simulink model "Turbine_model"  (R2023a)
settings: Solver=VariableStepAuto  StartTime=0.0  StopTime=10.0  RelTol=1e-3
values from neighbouring files (symbols this model uses):
  d_base = data_DF(13)    [find_dfig_state_initial_conditions.m]    (also in test_dfig.m = 5)
  d_Beta = 0    [dfig_smib_main.m]    (also in find_dfig_state_initial_conditions.m; test_dfig.m)
  d_bl = 40.05    [dfig_smib_main.m]    (also in find_dfig_state_initial_conditions.m; test_dfig.m)
  d_Cdc = 2    [dfig_smib_main.m]    (also in find_dfig_state_initial_conditions.m; test_dfig.m)
  d_Cf = 0.0150    (= 0.015)    [dfig_smib_main.m]    (also in find_dfig_state_initial_conditions.m = d_FLTR(6); test_dfig.m)
  d_ctg = 0.01    [dfig_smib_main.m]    (also in find_dfig_state_initial_conditions.m = data_DF(10); test_dfig.m)
  d_esd = -d_Kmrr.*d_ws.*(d_Lrr.*d_irq + d_Lm.*d_isq)    [find_dfig_state_initial_conditions.m]
  d_esq = d_Kmrr.*d_ws.*(d_Lrr.*d_ird + d_Lm.*d_isd)    [find_dfig_state_initial_conditions.m]
  d_iid = 0.0024    [dfig_smib_main.m]    (also in test_dfig.m)
  d_iiq = xdfig(:,7)    [find_dfig_state_initial_conditions.m]
  d_isd = 0.2454    [dfig_smib_main.m]    (also in find_dfig_state_initial_conditions.m = xdfig(:,2); test_dfig.m)
  d_isq = xdfig(:,1)    [find_dfig_state_initial_conditions.m]
  d_Kmrr = d_Lm/d_Lrr    (= 0.98517314418)    [dfig_smib_main.m]    (also in find_dfig_state_initial_conditions.m = d_Lm/d_Lrr; test_dfig.m)
  d_kopt = 1    [dfig_smib_main.m]    (also in find_dfig_state_initial_conditions.m = data_DF(8); test_dfig.m)
  d_ktg = 0.3    [dfig_smib_main.m]    (also in find_dfig_state_initial_conditions.m = data_DF(9); test_dfig.m)
  d_Lg = 0.0033    [dfig_smib_main.m]    (also in find_dfig_state_initial_conditions.m = d_FLTR(5); test_dfig.m)
  d_Li = 0.1667    [dfig_smib_main.m]    (also in find_dfig_state_initial_conditions.m = d_FLTR(4); test_dfig.m)
  d_Lm = 4    [dfig_smib_main.m]    (also in find_dfig_state_initial_conditions.m = data_DF(3); test_dfig.m)
  d_MSC_IL1_iv = 0.0389    [dfig_smib_main.m]    (also in test_dfig.m)
  d_MSC_IL1_ki = -3    [dfig_smib_main.m]    (also in find_dfig_state_initial_conditions.m; test_dfig.m)
  d_MSC_IL1_kp = -0.23    [dfig_smib_main.m]    (also in find_dfig_state_initial_conditions.m; test_dfig.m)
  d_MSC_IL2_ki = -3    [dfig_smib_main.m]    (also in find_dfig_state_initial_conditions.m; test_dfig.m)
  d_MSC_IL2_kp = -0.23    [dfig_smib_main.m]    (also in find_dfig_state_initial_conditions.m; test_dfig.m)
  d_MSC_OL1_iv = -0.8927    [dfig_smib_main.m]    (also in test_dfig.m)
  d_MSC_OL1_ki = -60    [dfig_smib_main.m]    (also in find_dfig_state_initial_conditions.m; test_dfig.m)
  d_MSC_OL1_kp = 0    [dfig_smib_main.m]    (also in find_dfig_state_initial_conditions.m; test_dfig.m)
  d_MSC_OL2_ki = 90    [dfig_smib_main.m]    (also in find_dfig_state_initial_conditions.m; test_dfig.m)
  d_MSC_OL2_kp = 0    [dfig_smib_main.m]    (also in find_dfig_state_initial_conditions.m; test_dfig.m)
  d_Qs = 0.1    [dfig_smib_main.m]    (also in find_dfig_state_initial_conditions.m = Qdfiq; test_dfig.m)
  d_R1 = d_Rs + d_R2    (= 0.0103381136821)    [dfig_smib_main.m]    (also in find_dfig_state_initial_conditions.m = d_Rs + d_R2; test_dfig.m)
  d_R2 = d_Kmrr^2*d_Rr    (= 0.00533811368208)    [dfig_smib_main.m]    (also in find_dfig_state_initial_conditions.m = d_Kmrr^2*d_Rr; test_dfig.m)
  d_Rc = 0.7333    [dfig_smib_main.m]    (also in find_dfig_state_initial_conditions.m = d_FLTR(3); test_dfig.m)
  d_Rg = 0.0    (= 0)    [dfig_smib_main.m]    (also in find_dfig_state_initial_conditions.m; test_dfig.m)
  d_Ri = 0.0    (= 0)    [dfig_smib_main.m]    (also in find_dfig_state_initial_conditions.m; test_dfig.m)
  d_Tr = d_Lrr/d_Rr    [find_dfig_state_initial_conditions.m]
  d_Ts = 0.9385    [dfig_smib_main.m]    (also in find_dfig_state_initial_conditions.m = dTg; test_dfig.m)
  d_vcq = 0.9837    [dfig_smib_main.m]    (also in find_dfig_state_initial_conditions.m = xdfig(:,13); test_dfig.m)
  d_VDC = 1.5    [dfig_smib_main.m]    (also in test_dfig.m)
  d_vrd = 0.0154    [dfig_smib_main.m]    (also in test_dfig.m)
  d_vrq = 0.0357    [dfig_smib_main.m]    (also in test_dfig.m)
  d_vw = 14.5316    [dfig_smib_main.m]    (also in test_dfig.m)
  d_welb = 2*pi*50    (= 314.159265359)    [find_dfig_state_initial_conditions.m]    (also in test_dfig.m)
  d_ws = 1.0    (= 1)    [find_dfig_state_initial_conditions.m]    (also in test_dfig.m = 314.159265359)
  d_wtrated = 3.0337    [dfig_smib_main.m]    (also in find_dfig_state_initial_conditions.m; test_dfig.m)
  d_Xm = d_Lm    (= 4)    [dfig_smib_main.m]    (also in find_dfig_state_initial_conditions.m = d_Lm; test_dfig.m)
  rho = 1.225    [dfig_smib_main.m]    (also in find_dfig_state_initial_conditions.m; test_dfig.m)
undefined symbols (not defined in the file or in its folder): d_Lsd, d_p, d_vdc, d_w, d_wb
settings Model: Creator=rufar  LastModifiedBy=rufar

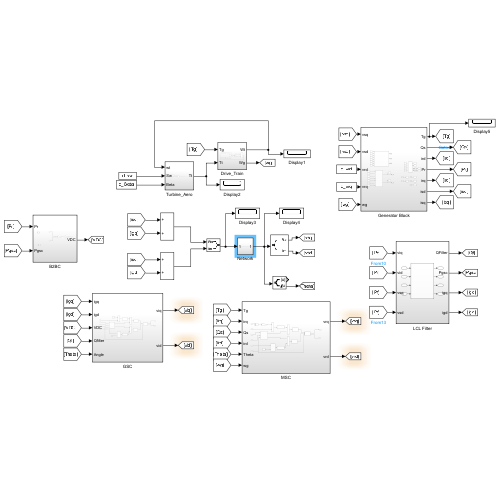
[thumbnail: Simulink's stored preview of the top-level diagram]
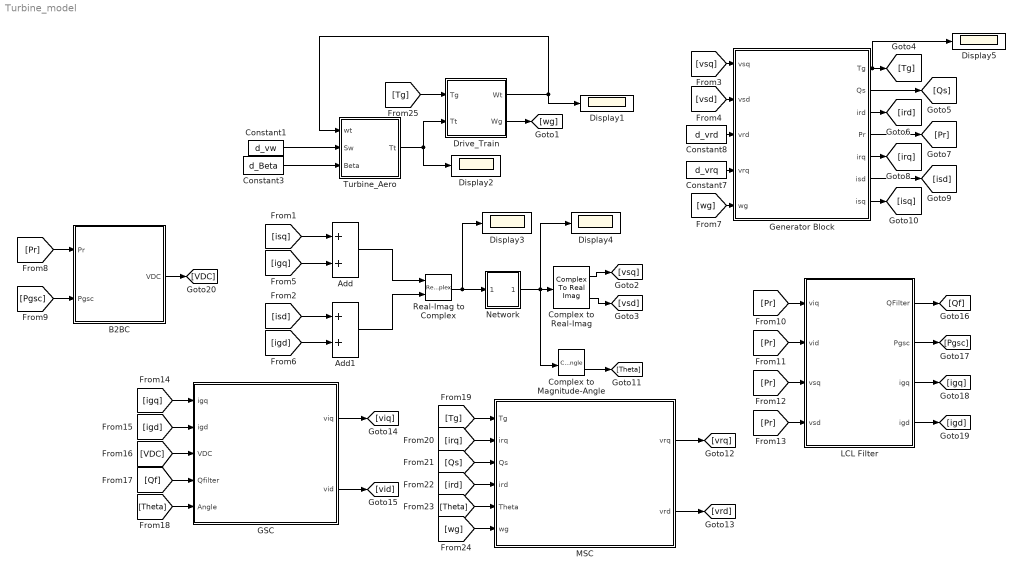
== system Turbine_model ==
  Add : Sum
  Add1 : Sum
  B2BC : Subsystem
  Complex to Magnitude-Angle : ComplexToMagnitudeAngle
  Complex to Real-Imag : ComplexToRealImag
  Constant1 : Constant  Value=d_vw
  Constant3 : Constant  Value=d_Beta
  Constant7 : Constant  Value=d_vrq
  Constant8 : Constant  Value=d_vrd
  Display{1..5} (5 alike) : Scope
  Drive_Train : Subsystem
  GSC : Subsystem
  Generator Block : Subsystem
  LCL Filter : Subsystem
  MSC : Subsystem
  Network : Subsystem
  Real-Imag to Complex : RealImagToComplex
  Turbine_Aero : Subsystem
  wires:
  Constant1/1 -> Turbine_Aero/2(Sw)
  Constant3/1 -> Turbine_Aero/3(Beta)
  Drive_Train/1(Wt) -> Display1/1, Turbine_Aero/1(wt)
  [Tg] -> Drive_Train/1(Tg)
  Drive_Train/2(Wg) -> [wg]
  Turbine_Aero/1(Tt) -> Drive_Train/2(Tt), Display2/1
  [igq] -> Add/2
  [igd] -> Add1/2
  Add/1 -> Real-Imag to Complex/1
  Add1/1 -> Real-Imag to Complex/2
  Real-Imag to Complex/1 -> Network/1(In1), Display3/1
  Complex to Real-Imag/1 -> [vsq]
  Complex to Real-Imag/2 -> [vsd]
  [isq] -> Add/1
  [isd] -> Add1/1
  [vsq] -> Generator Block/1(vsq)
  [vsd] -> Generator Block/2(vsd)
  [wg] -> Generator Block/5(wg)
  Constant7/1 -> Generator Block/4(vrq)
  Constant8/1 -> Generator Block/3(vrd)
  Generator Block/1(Tg) -> Display5/1, [Tg]
  Generator Block/2(Qs) -> [Qs]
  Generator Block/3(ird) -> [ird]
  Generator Block/4(Pr) -> [Pr]
  Generator Block/5(irq) -> [irq]
  Generator Block/6(isd) -> [isd]
  Generator Block/7(isq) -> [isq]
  Network/1(Out1) -> Complex to Magnitude-Angle/1, Display4/1, Complex to Real-Imag/1
  Complex to Magnitude-Angle/2 -> [Theta]
  [Pr] -> B2BC/1(Pr)
  [Pgsc] -> B2BC/2(Pgsc)
  [Pr] -> LCL Filter/1(viq)
  [Pr] -> LCL Filter/2(vid)
  [Pr] -> LCL Filter/3(vsq)
  [Pr] -> LCL Filter/4(vsd)
  [igq] -> GSC/1(igq)
  [igd] -> GSC/2(igd)
  [VDC] -> GSC/3(VDC)
  [Qf] -> GSC/4(Qfilter)
  [Theta] -> GSC/5(Angle)
  [Tg] -> MSC/1(Tg)
  [irq] -> MSC/2(irq)
  [Qs] -> MSC/3(Qs)
  [ird] -> MSC/4(ird)
  [Theta] -> MSC/5(Theta)
  [wg] -> MSC/6(wg)
  MSC/1(vrq) -> [vrq]
  MSC/2(vrd) -> [vrd]
  GSC/2(vid) -> [vid]
  GSC/1(viq) -> [viq]
  LCL Filter/1(QFilter) -> [Qf]
  LCL Filter/3(igq) -> [igq]
  LCL Filter/4(igd) -> [igd]
  LCL Filter/2(Pgsc) -> [Pgsc]
  B2BC/1(VDC) -> [VDC]

== system Turbine_model/B2BC ==
  Pr : Inport
  Pgsc : Inport  Port=2
  Add : Sum
  Add1 : Sum  Inputs=+-
  Gain : Gain  Gain=d_Cdc/d_p
  Gain1 : Gain  Gain=1/d_vdc
  Product : Product
  VDC : Outport
  wires:
  Gain/1 -> VDC/1
  Pr/1 -> Add1/1
  Pgsc/1 -> Add1/2
  Add1/1 -> Gain1/1
  Gain1/1 -> Gain/1

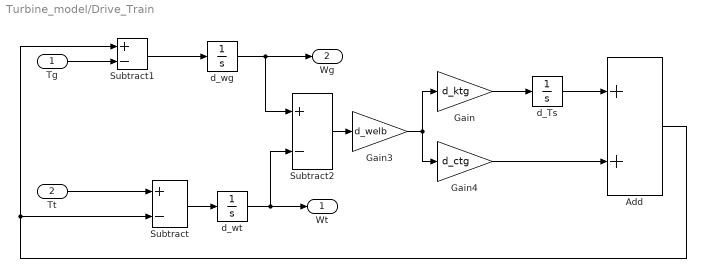
== system Turbine_model/Drive_Train ==
  Tg : Inport
  Tt : Inport  Port=2
  Add : Sum
  Gain : Gain  Gain=d_ktg
  Gain3 : Gain  Gain=d_welb
  Gain4 : Gain  Gain=d_ctg
  Subtract : Sum  Inputs=+-
  Subtract1 : Sum  Inputs=+-
  Subtract2 : Sum  Inputs=+-
  d_Ts : Integrator  InitialCondition=d_Ts
  d_wg : Integrator
  d_wt : Integrator
  Wt : Outport
  Wg : Outport  Port=2
  wires:
  Subtract1/1 -> d_wg/1
  Tg/1 -> Subtract1/2
  Gain3/1 -> Gain/1, Gain4/1
  d_wt/1 -> Wt/1, Subtract2/2
  Add/1 -> Subtract1/1, Subtract/2
  d_Ts/1 -> Add/1
  d_wg/1 -> Wg/1, Subtract2/1
  Gain/1 -> d_Ts/1
  Subtract2/1 -> Gain3/1
  Tt/1 -> Subtract/1
  Subtract/1 -> d_wt/1
  Gain4/1 -> Add/2

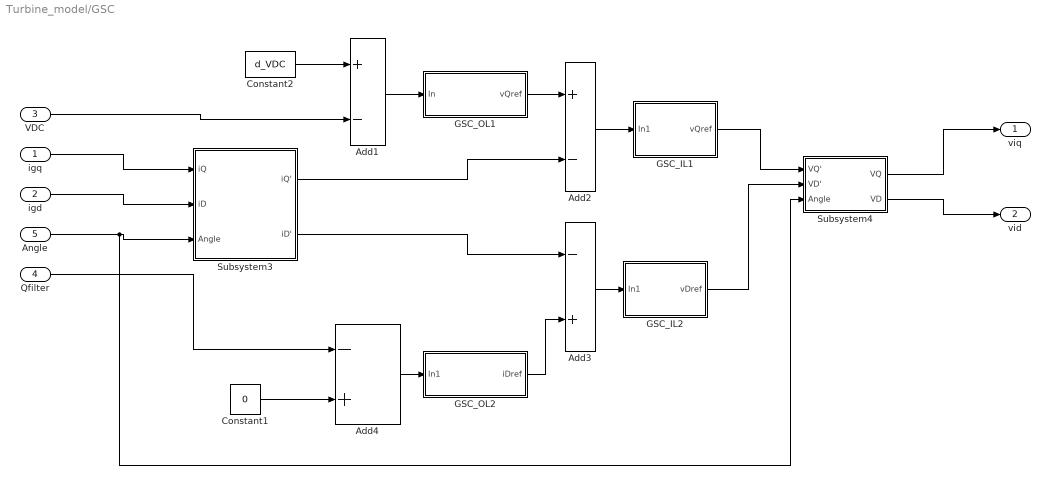
== system Turbine_model/GSC ==
  igq : Inport
  igd : Inport  Port=2
  VDC : Inport  Port=3
  Qfilter : Inport  Port=4
  Angle : Inport  Port=5
  Add1 : Sum  Inputs=+-
  Add2 : Sum  Inputs=+-
  Add3 : Sum  Inputs=-+
  Add4 : Sum  Inputs=-+
  Constant1 : Constant  Value=0
  Constant2 : Constant  Value=d_VDC
  GSC_IL1 : Subsystem
  GSC_IL2 : Subsystem
  GSC_OL1 : Subsystem
  GSC_OL2 : Subsystem
  Subsystem3 : Subsystem
  Subsystem4 : Subsystem
  viq : Outport
  vid : Outport  Port=2
  wires:
  Add2/1 -> GSC_IL1/1(In1)
  Constant1/1 -> Add4/2
  GSC_IL2/1(vDref) -> Subsystem4/2(VD')
  GSC_OL2/1(iDref) -> Add3/2
  Subsystem3/2(iD') -> Add3/1
  Add3/1 -> GSC_IL2/1(In1)
  GSC_IL1/1(vQref) -> Subsystem4/1(VQ')
  Add4/1 -> GSC_OL2/1(In1)
  Subsystem3/1(iQ') -> Add2/2
  GSC_OL1/1(vQref) -> Add2/1
  Add1/1 -> GSC_OL1/1(In)
  Constant2/1 -> Add1/1
  Qfilter/1 -> Add4/1
  VDC/1 -> Add1/2
  igq/1 -> Subsystem3/1(iQ)
  igd/1 -> Subsystem3/2(iD)
  Angle/1 -> Subsystem4/3(Angle), Subsystem3/3(Angle)
  Subsystem4/1(VQ) -> viq/1
  Subsystem4/2(VD) -> vid/1

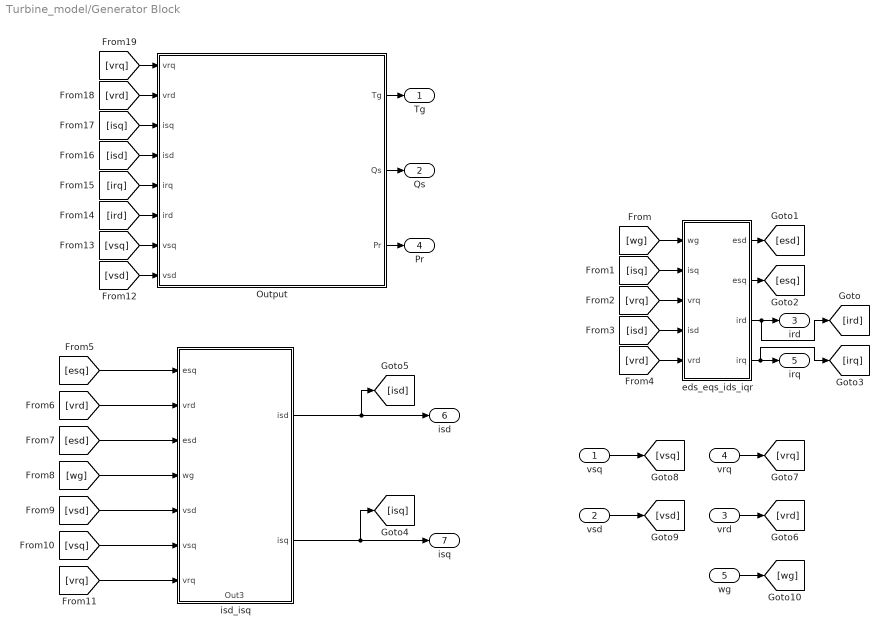
== system Turbine_model/Generator Block ==
  vsq : Inport
  vsd : Inport  Port=2
  vrd : Inport  Port=3
  vrq : Inport  Port=4
  wg : Inport  Port=5
  Output : Subsystem
  eds_eqs_ids_iqr : Subsystem
  isd_isq : Subsystem
      settings: PortSchema="{\"entries\":[{\"content\":{\"sides\":[{\"content\":{\"connectorIds\":[\"In1\",\"In2\",\"In3\",\"In4\",\"In5\",\"In6\",\"In7\"]},\"type\":\"ConnectorPlacement.EquallySpacedRectSide\",\"uuid\":\"c5511185-da93-4ae8-88f6-29fd087d6847\"},{\"content\":{\"connectorIds\":[\"Out1\",\"Out2\"],\"side\":\"RIGHT\"},\"type\":\"ConnectorPlacement.EquallySpacedRectSide\",\"uuid\":\"8a51c219-b932-42a4-96d0-f80c9d1d2533\"},{\"content\":{\"side\":\"TOP\"},\"type\":\"ConnectorPlacement.EquallySpacedRectSide\",\"uuid\":\"7f9cc9f4-8f0b-466b-9f07-e1686915bf69\"},{\"content\":{\"connectorIds\":[\"Out3\"],\"side\":\"BOTTOM\"},\"type\":\"ConnectorPlacement.EquallySpacedRectSide\",\"uuid\":\"e11d6ee8-9751-46c5-ba7a-4a49ef168c79\"}]},\"type\":\"ConnectorPlacement.EquallySpacedConnector\",\"uuid\":\"445fd2cf-43b7-4f11-a009-da067b61af35\"}],\"packageUris\":[\"http://schema.mathworks.com/mf0/Connector/R2020b\"],\"version\":\"1.0\"}"
  Tg : Outport
  Qs : Outport  Port=2
  ird : Outport  Port=3
  Pr : Outport  Port=4
  irq : Outport  Port=5
  isd : Outport  Port=6
  isq : Outport  Port=7
  wires:
  [isd] -> eds_eqs_ids_iqr/4(isd)
  [esq] -> isd_isq/1(esq)
  [wg] -> isd_isq/4(wg)
  [vrq] -> isd_isq/7(vrq)
  Output/1(Tg) -> Tg/1
  isd_isq/1(isd) -> [isd], isd/1
  isd_isq/2("isq ") -> [isq], isq/1
  [irq] -> Output/5(irq)
  [vrd] -> isd_isq/2(vrd)
  Output/3(Pr) -> Pr/1
  eds_eqs_ids_iqr/1(esd) -> [esd]
  [vrq] -> eds_eqs_ids_iqr/3(vrq)
  [isd] -> Output/4(isd)
  eds_eqs_ids_iqr/4(irq) -> [irq], irq/1
  [vsd] -> isd_isq/5(vsd)
  [esd] -> isd_isq/3(esd)
  [isq] -> eds_eqs_ids_iqr/2(isq)
  [vrd] -> eds_eqs_ids_iqr/5(vrd)
  [vsq] -> isd_isq/6(vsq)
  eds_eqs_ids_iqr/2(esq) -> [esq]
  [isq] -> Output/3(isq)
  [ird] -> Output/6(ird)
  [vsq] -> Output/7(vsq)
  [vsd] -> Output/8(vsd)
  [vrd] -> Output/2(vrd)
  Output/2(Qs) -> Qs/1
  [vrq] -> Output/1(vrq)
  [wg] -> eds_eqs_ids_iqr/1(wg)
  eds_eqs_ids_iqr/3(ird) -> [ird], ird/1
  vsq/1 -> [vsq]
  vsd/1 -> [vsd]
  vrd/1 -> [vrd]
  vrq/1 -> [vrq]
  wg/1 -> [wg]

== system Turbine_model/LCL Filter ==
  viq : Inport
  vid : Inport  Port=2
  vsq : Inport  Port=3
  vsd : Inport  Port=4
  LCL Filter : Subsystem
  QFilter : Outport
  Pgsc : Outport  Port=2
  igq : Outport  Port=3
  igd : Outport  Port=4
  wires:
  viq/1 -> LCL Filter/1(viq)
  LCL Filter/2(Pgsc) -> Pgsc/1
  vsd/1 -> LCL Filter/4(vsd)
  vsq/1 -> LCL Filter/3(vsq)
  vid/1 -> LCL Filter/2(vid)
  LCL Filter/1(QFilter) -> QFilter/1
  LCL Filter/3(igq) -> igq/1
  LCL Filter/4(igd) -> igd/1

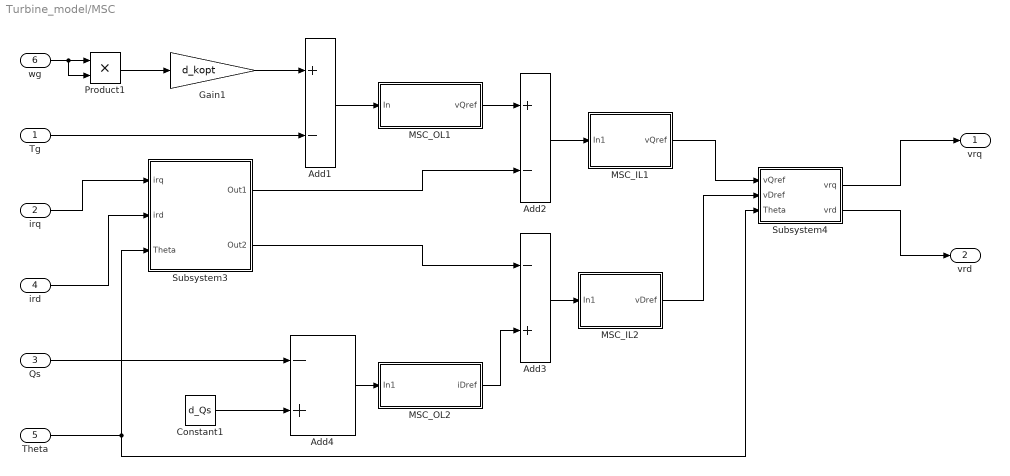
== system Turbine_model/MSC ==
  Tg : Inport
  irq : Inport  Port=2
  Qs : Inport  Port=3
  ird : Inport  Port=4
  Theta : Inport  Port=5
  wg : Inport  Port=6
  Add1 : Sum  Inputs=+-
  Add2 : Sum  Inputs=+-
  Add3 : Sum  Inputs=-+
  Add4 : Sum  Inputs=-+
  Constant1 : Constant  Value=d_Qs
  Gain1 : Gain  Gain=d_kopt
  MSC_IL1 : Subsystem
  MSC_IL2 : Subsystem
  MSC_OL1 : Subsystem
  MSC_OL2 : Subsystem
  Product1 : Product
  Subsystem3 : Subsystem
  Subsystem4 : Subsystem
  vrq : Outport
  vrd : Outport  Port=2
  wires:
  wg/1 -> Product1/2, Product1/1
  Product1/1 -> Gain1/1
  Gain1/1 -> Add1/1
  Tg/1 -> Add1/2
  Add1/1 -> MSC_OL1/1(In)
  MSC_OL1/1(vQref) -> Add2/1
  irq/1 -> Subsystem3/1(irq)
  ird/1 -> Subsystem3/2(ird)
  Theta/1 -> Subsystem4/3(Theta), Subsystem3/3(Theta)
  Subsystem3/1(Out1) -> Add2/2
  Qs/1 -> Add4/1
  Constant1/1 -> Add4/2
  Subsystem4/1(vrq) -> vrq/1
  Subsystem3/2(Out2) -> Add3/1
  Subsystem4/2(vrd) -> vrd/1
  MSC_IL2/1(vDref) -> Subsystem4/2(vDref)
  MSC_IL1/1(vQref) -> Subsystem4/1(vQref)
  Add3/1 -> MSC_IL2/1(In1)
  MSC_OL2/1(iDref) -> Add3/2
  Add2/1 -> MSC_IL1/1(In1)
  Add4/1 -> MSC_OL2/1(In1)

== system Turbine_model/Network ==
  In1 : Inport
  Out1 : Outport
  wires:
  In1/1 -> Out1/1

== system Turbine_model/Turbine_Aero ==
  wt : Inport
  Sw : Inport  Port=2
  Beta : Inport  Port=3
  Subsystem : Subsystem
  Tt : Outport
  wires:
  Beta/1 -> Subsystem/3(Beta)
  Subsystem/1(Tt) -> Tt/1
  Sw/1 -> Subsystem/2(Sw)
  wt/1 -> Subsystem/1(wt)

== system Turbine_model/GSC/GSC_IL1 ==
  In1 : Inport
  Gain1 : Gain  Gain=d_MSC_IL1_ki
  Gain2 : Gain  Gain=d_MSC_IL1_kp
  Sum : Sum
  d_MSC_IL1_lv : Integrator  InitialCondition=d_MSC_IL1_iv
  vQref : Outport
  wires:
  In1/1 -> Gain2/1, Gain1/1
  Gain1/1 -> d_MSC_IL1_lv/1
  Gain2/1 -> Sum/2
  Sum/1 -> vQref/1
  d_MSC_IL1_lv/1 -> Sum/1

== system Turbine_model/GSC/GSC_IL2 ==
  In1 : Inport
  Gain1 : Gain  Gain=d_MSC_IL2_ki
  Gain2 : Gain  Gain=d_MSC_IL2_kp
  Sum : Sum
  d_MSC_IL2_lv : Integrator  InitialCondition=d_MSC_IL1_iv
  vDref : Outport
  wires:
  d_MSC_IL2_lv/1 -> Sum/1
  Gain2/1 -> Sum/2
  Sum/1 -> vDref/1
  Gain1/1 -> d_MSC_IL2_lv/1
  In1/1 -> Gain2/1, Gain1/1

== system Turbine_model/GSC/GSC_OL1 ==
  In : Inport
  Gain1 : Gain  Gain=d_MSC_OL1_ki
  Gain2 : Gain  Gain=d_MSC_OL1_kp
  Sum : Sum
  d_MSC_OL1_lv : Integrator  InitialCondition=d_MSC_OL1_iv
  vQref : Outport
  wires:
  Gain1/1 -> d_MSC_OL1_lv/1
  d_MSC_OL1_lv/1 -> Sum/1
  Gain2/1 -> Sum/2
  Sum/1 -> vQref/1
  In/1 -> Gain2/1, Gain1/1

== system Turbine_model/GSC/GSC_OL2 ==
  In1 : Inport
  Gain1 : Gain  Gain=d_MSC_OL2_ki
  Gain2 : Gain  Gain=d_MSC_OL2_kp
  Sum : Sum
  d_MSC_OL2_lv : Integrator  InitialCondition=d_MSC_OL1_iv
  iDref : Outport
  wires:
  In1/1 -> Gain2/1, Gain1/1
  Gain1/1 -> d_MSC_OL2_lv/1
  Gain2/1 -> Sum/2
  Sum/1 -> iDref/1
  d_MSC_OL2_lv/1 -> Sum/1

== system Turbine_model/GSC/Subsystem3 ==
  iQ : Inport
  iD : Inport  Port=2
  Angle : Inport  Port=3
  iQ' : Outport
  iD' : Outport  Port=2
  wires:
  iQ/1 -> iQ'/1

== system Turbine_model/GSC/Subsystem4 ==
  VQ' : Inport
  VD' : Inport  Port=2
  Angle : Inport  Port=3
  VQ : Outport
  VD : Outport  Port=2
  wires:
  VQ'/1 -> VD/1

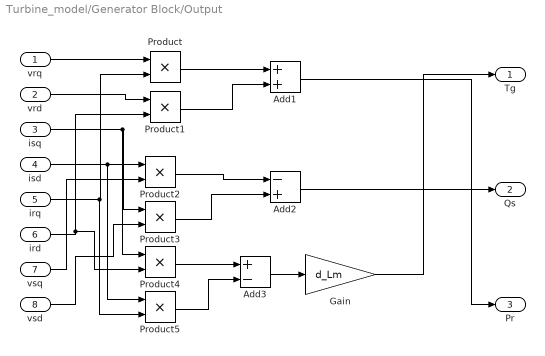
== system Turbine_model/Generator Block/Output ==
  vrq : Inport
  vrd : Inport  Port=2
  isq : Inport  Port=3
  isd : Inport  Port=4
  irq : Inport  Port=5
  ird : Inport  Port=6
  vsq : Inport  Port=7
  vsd : Inport  Port=8
  Add1 : Sum
  Add2 : Sum  Inputs=-+
  Add3 : Sum  Inputs=+-
  Gain : Gain  Gain=d_Lm
  Product{,1..5} (6 alike) : Product
  Tg : Outport
  Qs : Outport  Port=2
  Pr : Outport  Port=3
  wires:
  vrq/1 -> Product/1
  vrd/1 -> Product1/1
  isq/1 -> Product4/1, Product3/1
  isd/1 -> Product2/1, Product5/1
  irq/1 -> Product5/2, Product/2
  ird/1 -> Product4/2, Product1/2
  Product/1 -> Add1/1
  Product1/1 -> Add1/2
  Add1/1 -> Pr/1
  Product3/1 -> Add2/2
  vsq/1 -> Product2/2
  Product2/1 -> Add2/1
  vsd/1 -> Product3/2
  Add2/1 -> Qs/1
  Add3/1 -> Gain/1
  Gain/1 -> Tg/1
  Product5/1 -> Add3/2
  Product4/1 -> Add3/1

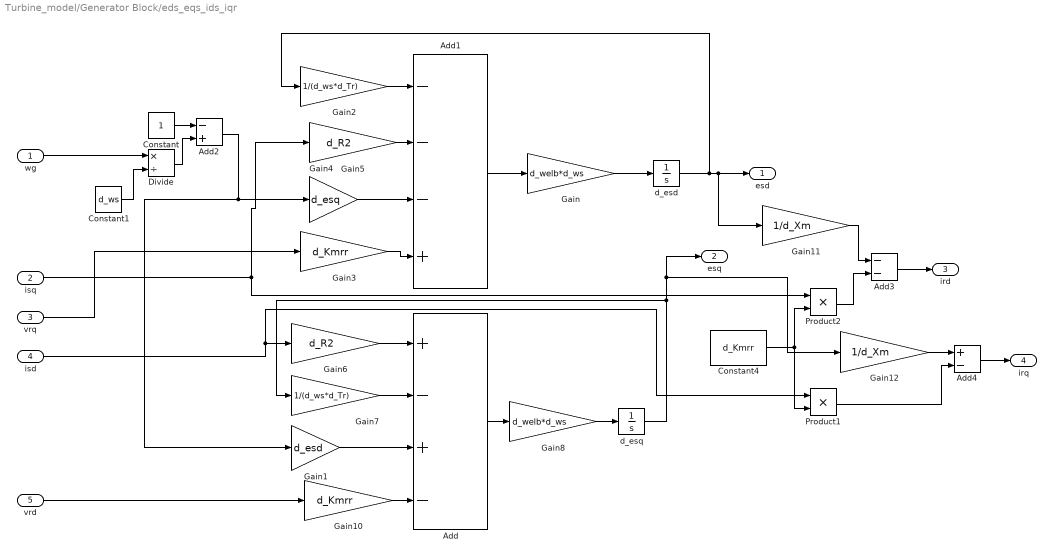
== system Turbine_model/Generator Block/eds_eqs_ids_iqr ==
  wg : Inport
  isq : Inport  Port=2
  vrq : Inport  Port=3
  isd : Inport  Port=4
  vrd : Inport  Port=5
  Add : Sum  Inputs=+-+-
  Add1 : Sum  Inputs=---+
  Add2 : Sum  Inputs=-+
  Add3 : Sum  Inputs=--
  Add4 : Sum  Inputs=+-
  Constant : Constant
  Constant1 : Constant  Value=d_ws
  Constant4 : Constant  Value=d_Kmrr
  Divide : Product  Inputs=*/
  Gain : Gain  Gain=d_welb*d_ws
  Gain1 : Gain  Gain=d_esd
  Gain10 : Gain  Gain=d_Kmrr
  Gain11 : Gain  Gain=1/d_Xm
  Gain12 : Gain  Gain=1/d_Xm
  Gain2 : Gain  Gain=1/(d_ws*d_Tr)
  Gain3 : Gain  Gain=d_Kmrr
  Gain4 : Gain  Gain=d_esq
  Gain5 : Gain  Gain=d_R2
  Gain6 : Gain  Gain=d_R2
  Gain7 : Gain  Gain=1/(d_ws*d_Tr)
  Gain8 : Gain  Gain=d_welb*d_ws
  Product1 : Product
  Product2 : Product
  d_esd : Integrator  InitialCondition=d_esd
  d_esq : Integrator  InitialCondition=d_esq
  esd : Outport
  esq : Outport  Port=2
  ird : Outport  Port=3
  irq : Outport  Port=4
  wires:
  Add1/1 -> Gain/1
  isd/1 -> Product1/1, Gain6/1
  Product1/1 -> Add4/2
  Gain2/1 -> Add1/1
  Gain6/1 -> Add/1
  Product2/1 -> Add3/2
  Constant4/1 -> Product2/2, Product1/2
  Gain3/1 -> Add1/4
  d_esd/1 -> Gain2/1, esd/1, Gain11/1
  d_esq/1 -> Gain7/1, esq/1, Gain12/1
  Add4/1 -> irq/1
  Gain/1 -> d_esd/1
  Gain11/1 -> Add3/1
  Gain7/1 -> Add/2
  Gain8/1 -> d_esq/1
  Gain5/1 -> Add1/2
  Gain10/1 -> Add/4
  isq/1 -> Product2/1, Gain5/1
  Add/1 -> Gain8/1
  Add3/1 -> ird/1
  Gain12/1 -> Add4/1
  vrq/1 -> Gain3/1
  vrd/1 -> Gain10/1
  Constant/1 -> Add2/1
  wg/1 -> Divide/1
  Constant1/1 -> Divide/2
  Divide/1 -> Add2/2
  Add2/1 -> Gain1/1, Gain4/1
  Gain1/1 -> Add/3
  Gain4/1 -> Add1/3

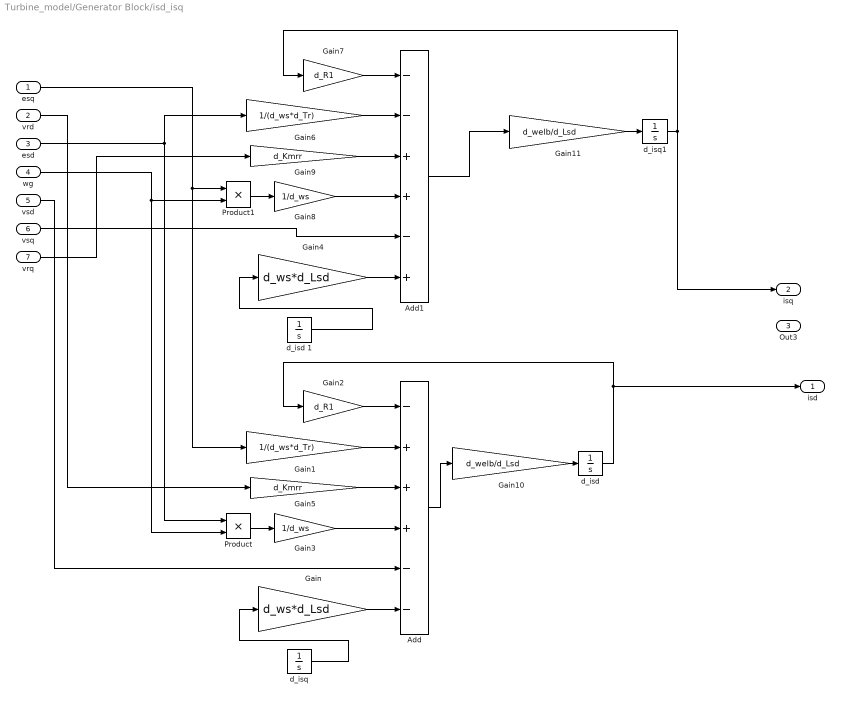
== system Turbine_model/Generator Block/isd_isq ==
  esq : Inport
  vrd : Inport  Port=2
  esd : Inport  Port=3
  wg : Inport  Port=4
  vsd : Inport  Port=5
  vsq : Inport  Port=6
  vrq : Inport  Port=7
  Add : Sum  Inputs=-+++--
  Add1 : Sum  Inputs=--++-+
  Gain : Gain  Gain=d_ws*d_Lsd
  Gain1 : Gain  Gain=1/(d_ws*d_Tr)
  Gain10 : Gain  Gain=d_welb/d_Lsd
  Gain11 : Gain  Gain=d_welb/d_Lsd
  Gain2 : Gain  Gain=d_R1
  Gain3 : Gain  Gain=1/d_ws
  Gain4 : Gain  Gain=d_ws*d_Lsd
  Gain5 : Gain  Gain=d_Kmrr
  Gain6 : Gain  Gain=1/(d_ws*d_Tr)
  Gain7 : Gain  Gain=d_R1
  Gain8 : Gain  Gain=1/d_ws
  Gain9 : Gain  Gain=d_Kmrr
  Product : Product
  Product1 : Product
  d_isd : Integrator  InitialCondition=d_isd
  d_isd 1 : Integrator  InitialCondition=d_isd
  "d_isq " : Integrator  InitialCondition=d_isq
  d_isq1 : Integrator  InitialCondition=d_isq
  isd : Outport
  "isq " : Outport  Port=2
  Out3 : Outport  Port=3
  wires:
  esd/1 -> Product/1, Gain6/1
  Gain1/1 -> Add/2
  vsq/1 -> Add1/5
  d_isd 1/1 -> Gain4/1
  Add/1 -> Gain10/1
  d_isq1/1 -> "isq "/1, Gain7/1
  Gain8/1 -> Add1/4
  Product1/1 -> Gain8/1
  Gain4/1 -> Add1/6
  Gain9/1 -> Add1/3
  Gain7/1 -> Add1/1
  wg/1 -> Product1/2, Product/2
  Add1/1 -> Gain11/1
  Gain6/1 -> Add1/2
  vrq/1 -> Gain9/1
  vrd/1 -> Gain5/1
  esq/1 -> Product1/1, Gain1/1
  vsd/1 -> Add/5
  d_isd/1 -> isd/1, Gain2/1
  Gain10/1 -> d_isd/1
  Gain2/1 -> Add/1
  Product/1 -> Gain3/1
  "d_isq "/1 -> Gain/1
  Gain11/1 -> d_isq1/1
  Gain/1 -> Add/6
  Gain5/1 -> Add/3
  Gain3/1 -> Add/4

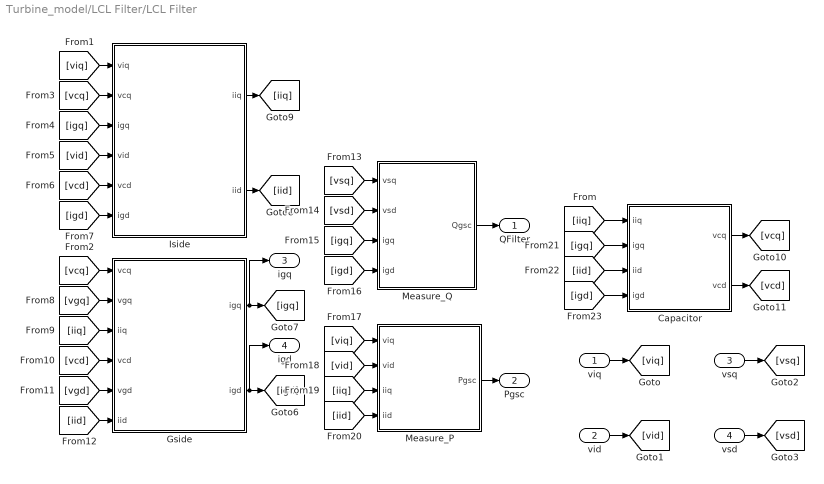
== system Turbine_model/LCL Filter/LCL Filter ==
  viq : Inport
  vid : Inport  Port=2
  vsq : Inport  Port=3
  vsd : Inport  Port=4
  Capacitor : Subsystem
  Gside : Subsystem
  Iside : Subsystem
  Measure_P : Subsystem
  Measure_Q : Subsystem
  QFilter : Outport
  Pgsc : Outport  Port=2
  igq : Outport  Port=3
  igd : Outport  Port=4
  wires:
  viq/1 -> [viq]
  vsq/1 -> [vsq]
  vsd/1 -> [vsd]
  vid/1 -> [vid]
  [viq] -> Iside/1(viq)
  [vcq] -> Iside/2(vcq)
  [igq] -> Iside/3(igq)
  [vid] -> Iside/4(vid)
  [vcd] -> Iside/5(vcd)
  [igd] -> Iside/6(igd)
  [vcq] -> Gside/1(vcq)
  [vgq] -> Gside/2(vgq)
  [iiq] -> Gside/3(iiq)
  [vcd] -> Gside/4(vcd)
  [vgd] -> Gside/5(vgd)
  [iid] -> Gside/6(iid)
  [vsq] -> Measure_Q/1(vsq)
  [vsd] -> Measure_Q/2(vsd)
  [igq] -> Measure_Q/3(igq)
  [igd] -> Measure_Q/4(igd)
  [viq] -> Measure_P/1(viq)
  [vid] -> Measure_P/2(vid)
  [iiq] -> Measure_P/3(iiq)
  [iid] -> Measure_P/4(iid)
  Measure_Q/1(Qgsc) -> QFilter/1
  Measure_P/1(Pgsc) -> Pgsc/1
  Iside/2(iid) -> [iid]
  Iside/1(iiq) -> [iiq]
  Gside/1(igq) -> igq/1, [igq]
  Gside/2(igd) -> igd/1, [igd]
  [iiq] -> Capacitor/1(iiq)
  [igq] -> Capacitor/2(igq)
  [igd] -> Capacitor/4(igd)
  [iid] -> Capacitor/3(iid)
  Capacitor/1(vcq) -> [vcq]
  Capacitor/2(vcd) -> [vcd]

== system Turbine_model/MSC/MSC_IL1 ==
  In1 : Inport
  Gain1 : Gain  Gain=d_MSC_IL1_ki
  Gain2 : Gain  Gain=d_MSC_IL1_kp
  Sum : Sum
  d_MSC_IL1_lv : Integrator  InitialCondition=d_MSC_IL1_iv
  vQref : Outport
  wires:
  In1/1 -> Gain2/1, Gain1/1
  Gain1/1 -> d_MSC_IL1_lv/1
  Gain2/1 -> Sum/2
  Sum/1 -> vQref/1
  d_MSC_IL1_lv/1 -> Sum/1

== system Turbine_model/MSC/MSC_IL2 ==
  In1 : Inport
  Gain1 : Gain  Gain=d_MSC_IL2_ki
  Gain2 : Gain  Gain=d_MSC_IL2_kp
  Sum : Sum
  d_MSC_IL2_lv : Integrator  InitialCondition=d_MSC_IL1_iv
  vDref : Outport
  wires:
  d_MSC_IL2_lv/1 -> Sum/1
  Gain2/1 -> Sum/2
  Sum/1 -> vDref/1
  Gain1/1 -> d_MSC_IL2_lv/1
  In1/1 -> Gain2/1, Gain1/1

== system Turbine_model/MSC/MSC_OL1 ==
  In : Inport
  Gain1 : Gain  Gain=d_MSC_OL1_ki
  Gain2 : Gain  Gain=d_MSC_OL1_kp
  Sum : Sum
  d_MSC_OL1_lv : Integrator  InitialCondition=d_MSC_OL1_iv
  vQref : Outport
  wires:
  Gain1/1 -> d_MSC_OL1_lv/1
  d_MSC_OL1_lv/1 -> Sum/1
  Gain2/1 -> Sum/2
  Sum/1 -> vQref/1
  In/1 -> Gain2/1, Gain1/1

== system Turbine_model/MSC/MSC_OL2 ==
  In1 : Inport
  Gain1 : Gain  Gain=d_MSC_OL2_ki
  Gain2 : Gain  Gain=d_MSC_OL2_kp
  Sum : Sum
  d_MSC_OL2_lv : Integrator  InitialCondition=d_MSC_OL1_iv
  iDref : Outport
  wires:
  In1/1 -> Gain2/1, Gain1/1
  Gain1/1 -> d_MSC_OL2_lv/1
  Gain2/1 -> Sum/2
  Sum/1 -> iDref/1
  d_MSC_OL2_lv/1 -> Sum/1

== system Turbine_model/MSC/Subsystem3 ==
  irq : Inport
  ird : Inport  Port=2
  Theta : Inport  Port=3
  Out1 : Outport
  Out2 : Outport  Port=2
  wires:
  irq/1 -> Out1/1

== system Turbine_model/MSC/Subsystem4 ==
  vQref : Inport
  vDref : Inport  Port=2
  Theta : Inport  Port=3
  vrq : Outport
  vrd : Outport  Port=2
  wires:
  vQref/1 -> vrd/1

== system Turbine_model/Turbine_Aero/Subsystem ==
  wt : Inport
  Sw : Inport  Port=2
  Beta : Inport  Port=3
  Constant2 : Constant  Value=0.5*rho*pi*d_bl^2
  Constant4 : Constant  Value=3
  Cp_Calc : Subsystem
  Divide : Product  Inputs=*/
  Divide1 : Product  Inputs=/*
  Gain : Gain  Gain=d_wtrated*d_bl
  Gain1 : Gain  Gain=1/(d_base*10^6)
  Math Function : Math  Operator=pow
  Product : Product  Inputs=3
  Tt : Outport
  wires:
  Constant4/1 -> Math Function/2
  Math Function/1 -> Product/3
  Divide/1 -> Cp_Calc/1(Lamba)
  Cp_Calc/1(Cp) -> Product/2
  Sw/1 -> Math Function/1, Divide/2
  Product/1 -> Gain1/1
  Gain/1 -> Divide/1
  Constant2/1 -> Product/1
  Gain1/1 -> Divide1/2
  wt/1 -> Divide1/1, Gain/1
  Beta/1 -> Cp_Calc/2(Beta)
  Divide1/1 -> Tt/1

== system Turbine_model/LCL Filter/LCL Filter/Capacitor ==
  iiq : Inport
  igq : Inport  Port=2
  iid : Inport  Port=3
  igd : Inport  Port=4
  Add1 : Sum  Inputs=+--
  Add2 : Sum  Inputs=+-+
  Gain1 : Gain  Gain=d_wb/d_Cf
  Gain2 : Gain  Gain=d_wb/d_Cf
  Gain3 : Gain  Gain=d_w*d_Cf
  Gain4 : Gain  Gain=d_w*d_Cf
  Integrator1 : Integrator  InitialCondition=d_vcq
  Integrator2 : Integrator  InitialCondition=d_vcq
  vcq : Outport
  vcd : Outport  Port=2
  wires:
  Add1/1 -> Gain1/1
  Gain1/1 -> Integrator1/1
  Integrator1/1 -> vcq/1, Gain4/1
  iiq/1 -> Add1/1
  igq/1 -> Add1/2
  Integrator2/1 -> Gain3/1, vcd/1
  Gain2/1 -> Integrator2/1
  Gain3/1 -> Add1/3
  Gain4/1 -> Add2/1
  iid/1 -> Add2/3
  igd/1 -> Add2/2
  Add2/1 -> Gain2/1

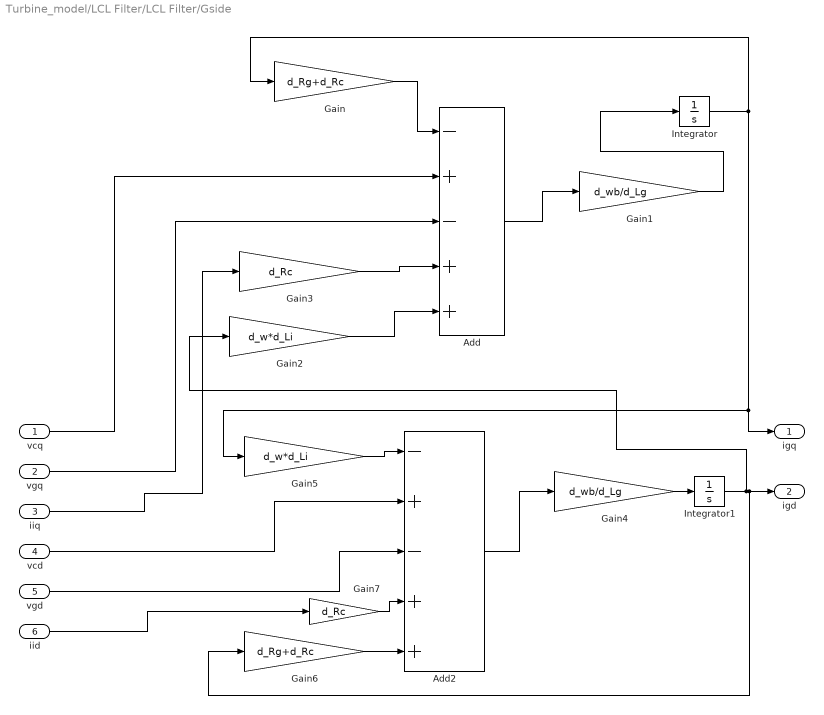
== system Turbine_model/LCL Filter/LCL Filter/Gside ==
  vcq : Inport
  vgq : Inport  Port=2
  iiq : Inport  Port=3
  vcd : Inport  Port=4
  vgd : Inport  Port=5
  iid : Inport  Port=6
  Add : Sum  Inputs=-+-++
  Add2 : Sum  Inputs=-+-++
  Gain : Gain  Gain=d_Rg+d_Rc
  Gain1 : Gain  Gain=d_wb/d_Lg
  Gain2 : Gain  Gain=d_w*d_Li
  Gain3 : Gain  Gain=d_Rc
  Gain4 : Gain  Gain=d_wb/d_Lg
  Gain5 : Gain  Gain=d_w*d_Li
  Gain6 : Gain  Gain=d_Rg+d_Rc
  Gain7 : Gain  Gain=d_Rc
  Integrator : Integrator  InitialCondition=d_iiq
  Integrator1 : Integrator  InitialCondition=d_iid
  igq : Outport
  igd : Outport  Port=2
  wires:
  Gain1/1 -> Integrator/1
  Gain7/1 -> Add2/4
  Gain3/1 -> Add/4
  Gain6/1 -> Add2/5
  iid/1 -> Gain7/1
  vcd/1 -> Add2/2
  Gain4/1 -> Integrator1/1
  iiq/1 -> Gain3/1
  Gain/1 -> Add/1
  vgd/1 -> Add2/3
  Add2/1 -> Gain4/1
  Integrator/1 -> Gain/1, Gain5/1, igq/1
  Add/1 -> Gain1/1
  vcq/1 -> Add/2
  Gain2/1 -> Add/5
  Gain5/1 -> Add2/1
  Integrator1/1 -> Gain2/1, Gain6/1, igd/1
  vgq/1 -> Add/3

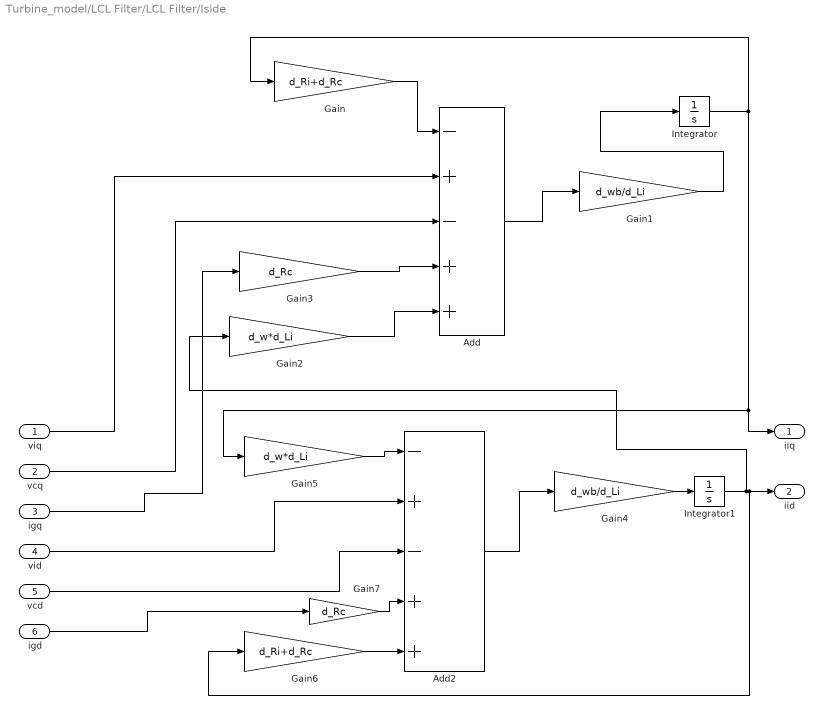
== system Turbine_model/LCL Filter/LCL Filter/Iside ==
  viq : Inport
  vcq : Inport  Port=2
  igq : Inport  Port=3
  vid : Inport  Port=4
  vcd : Inport  Port=5
  igd : Inport  Port=6
  Add : Sum  Inputs=-+-++
  Add2 : Sum  Inputs=-+-++
  Gain : Gain  Gain=d_Ri+d_Rc
  Gain1 : Gain  Gain=d_wb/d_Li
  Gain2 : Gain  Gain=d_w*d_Li
  Gain3 : Gain  Gain=d_Rc
  Gain4 : Gain  Gain=d_wb/d_Li
  Gain5 : Gain  Gain=d_w*d_Li
  Gain6 : Gain  Gain=d_Ri+d_Rc
  Gain7 : Gain  Gain=d_Rc
  Integrator : Integrator  InitialCondition=d_iiq
  Integrator1 : Integrator  InitialCondition=d_iid
  iiq : Outport
  iid : Outport  Port=2
  wires:
  vcq/1 -> Add/3
  viq/1 -> Add/2
  Add/1 -> Gain1/1
  Gain1/1 -> Integrator/1
  Integrator/1 -> Gain/1, Gain5/1, iiq/1
  Gain/1 -> Add/1
  Integrator1/1 -> Gain2/1, Gain6/1, iid/1
  Gain2/1 -> Add/5
  igq/1 -> Gain3/1
  Gain3/1 -> Add/4
  Gain4/1 -> Integrator1/1
  Add2/1 -> Gain4/1
  Gain5/1 -> Add2/1
  vid/1 -> Add2/2
  vcd/1 -> Add2/3
  Gain6/1 -> Add2/5
  igd/1 -> Gain7/1
  Gain7/1 -> Add2/4

== system Turbine_model/LCL Filter/LCL Filter/Measure_P ==
  viq : Inport
  vid : Inport  Port=2
  iiq : Inport  Port=3
  iid : Inport  Port=4
  Add : Sum
  Product : Product
  Product1 : Product
  Pgsc : Outport
  wires:
  iiq/1 -> Product/2
  viq/1 -> Product/1
  vid/1 -> Product1/1
  iid/1 -> Product1/2
  Product1/1 -> Add/2
  Product/1 -> Add/1
  Add/1 -> Pgsc/1

== system Turbine_model/LCL Filter/LCL Filter/Measure_Q ==
  vsq : Inport
  vsd : Inport  Port=2
  igq : Inport  Port=3
  igd : Inport  Port=4
  Add : Sum  Inputs=-+
  Product : Product
  Product1 : Product
  Qgsc : Outport
  wires:
  Add/1 -> Qgsc/1
  Product/1 -> Add/1
  Product1/1 -> Add/2
  igd/1 -> Product1/2
  vsd/1 -> Product1/1
  vsq/1 -> Product/1
  igq/1 -> Product/2

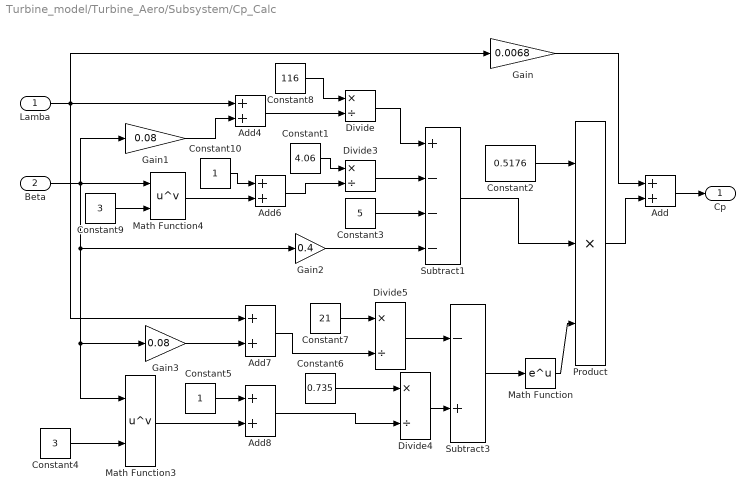
== system Turbine_model/Turbine_Aero/Subsystem/Cp_Calc ==
  Lamba : Inport
  Beta : Inport  Port=2
  Add{,4,6..8} (5 alike) : Sum
  Constant1 : Constant  Value=4.06
  Constant10 : Constant
  Constant2 : Constant  Value=0.5176
  Constant3 : Constant  Value=5
  Constant4 : Constant  Value=3
  Constant5 : Constant
  Constant6 : Constant  Value=0.735
  Constant7 : Constant  Value=21
  Constant8 : Constant  Value=116
  Constant9 : Constant  Value=3
  Divide{,3..5} (4 alike) : Product  Inputs=*/
  Gain : Gain  Gain=0.0068
  Gain1 : Gain  Gain=0.08
  Gain2 : Gain  Gain=0.4
  Gain3 : Gain  Gain=0.08
  Math Function : Math
  Math Function3 : Math  Operator=pow
  Math Function4 : Math  Operator=pow
  Product : Product  Inputs=3
  Subtract1 : Sum  Inputs=+---
  Subtract3 : Sum  Inputs=-+
  Cp : Outport
  wires:
  Lamba/1 -> Add4/1, Add7/1, Gain/1
  Gain1/1 -> Add4/2
  Add4/1 -> Divide/2
  Constant8/1 -> Divide/1
  Divide/1 -> Subtract1/1
  Subtract1/1 -> Product/2
  Product/1 -> Add/2
  Gain/1 -> Add/1
  Add/1 -> Cp/1
  Constant2/1 -> Product/1
  Math Function/1 -> Product/3
  Divide3/1 -> Subtract1/2
  Constant1/1 -> Divide3/1
  Add6/1 -> Divide3/2
  Constant3/1 -> Subtract1/3
  Gain2/1 -> Subtract1/4
  Beta/1 -> Math Function4/1, Math Function3/1, Gain3/1, Gain2/1, Gain1/1
  Gain3/1 -> Add7/2
  Constant4/1 -> Math Function3/2
  Math Function3/1 -> Add8/2
  Constant5/1 -> Add8/1
  Constant6/1 -> Divide4/1
  Add8/1 -> Divide4/2
  Divide4/1 -> Subtract3/2
  Divide5/1 -> Subtract3/1
  Constant7/1 -> Divide5/1
  Add7/1 -> Divide5/2
  Subtract3/1 -> Math Function/1
  Constant9/1 -> Math Function4/2
  Math Function4/1 -> Add6/2
  Constant10/1 -> Add6/1
